simulink model "nmpc_sim_ee"  (R2022a)
settings: Solver=ode45  StartTime=0.0  StopTime=7  FixedStep=0.1  RelTol=1e-3
values from neighbouring files (symbols this model uses):
  N = n + 6    [ctrl_comp.m]    (also in nmpc_ee_2DoF.m; nmpc_ee_6DoF.m; nmpc_ee_subtest.m; nmpc_joint.m)
  ref = struct()    [nmpc_ee_2DoF.m]    (also in nmpc_ee_6DoF.m; nmpc_ee_subtest.m)
  Tp = 5    [nmpc_ee_2DoF.m]    (also in nmpc_ee_6DoF.m; nmpc_ee_subtest.m; nmpc_joint.m = 10)
  Ts = 0.1    [nmpc_ee_2DoF.m]    (also in nmpc_ee_6DoF.m; nmpc_ee_subtest.m = 0.5; nmpc_joint.m = 0.2)
  xee0 = [xee0; zeros(3, 1)]    [nmpc_ee_2DoF.m]    (also in nmpc_ee_6DoF.m = [xee0; psi_ee]; nmpc_ee_subtest.m = xee_start)
libraries: mpclib x1
settings Model: Creator=charl  LastModifiedBy=charl

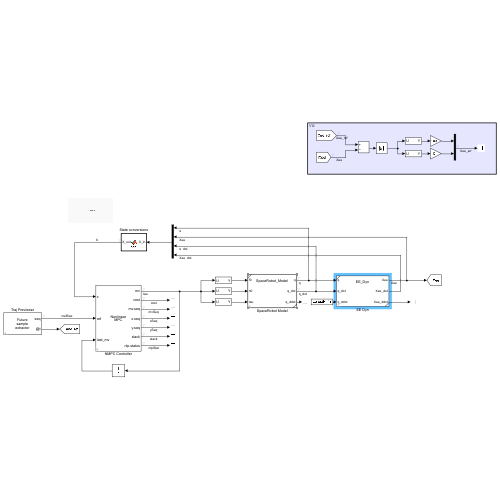
[thumbnail: Simulink's stored preview of the top-level diagram]
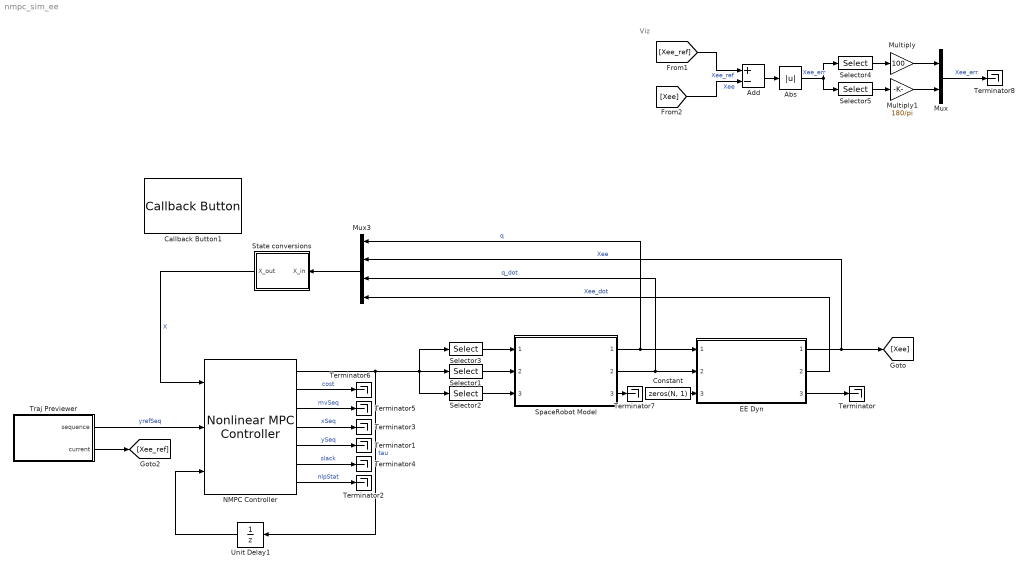
== system nmpc_sim_ee ==
  note: Viz
  Abs : Abs  SaturateOnIntegerOverflow=off
  Add : Sum  Inputs=+-
  Callback Button1 : CallbackButton  ButtonText=Animate results
      settings: ClickFcn=|
      | close all
      | try
      |     sr.animate(out.q, 'fps', 17, 'rate', 1);
      | catch
      |     close all
      | end
  Constant : Constant  Value=zeros(N, 1)
  EE Dyn : Subsystem  ReferencedSubsystem=EE_Dyn  spaceRobot=sr  Xee0=xee0.'
  Multiply : Gain  Gain=100
  Multiply1 : Gain  Gain=180/pi
  Mux : Mux  Inputs=2
  Mux3 : Mux
  NMPC Controller : mpclib/Nonlinear MPC Controller  SCDEnableBlockLinearizationSpecification=on  nlmpcobj=nlmpc_ee  UseObjectTs=on  TsControl=Ts  UseMEX=off  mexname=nlmpc_ee_SR6_mex  md_enabled=off  mvtarget_enabled=off  param_enabled=off  cost_enabled=on  mvseq_enabled=on  stateseq_enabled=on  ovseq_enabled=on  slack_enabled=on  status_enabled=on  ov_min=off  ov_max=off  mv_min=off  mv_max=off  mvrate_min=off  mvrate_max=off  state_min=off  state_max=off  ov_weight=off  mv_weight=off  mvrate_weight=off  ecr_weight=off  nlp_initialize=off
  Selector1 : Selector  IndexOptions=Index vector (dialog)  Indices=[4:6]  OutputSizes=1
  Selector2 : Selector  IndexOptions=Index vector (dialog)  Indices=[7:N]  OutputSizes=1
  Selector3 : Selector  IndexOptions=Index vector (dialog)  Indices=[1:3]  OutputSizes=1
  Selector4 : Selector  IndexOptions=Index vector (dialog)  Indices=[1:3]  OutputSizes=1
  Selector5 : Selector  IndexOptions=Index vector (dialog)  Indices=[4:6]  OutputSizes=1
  SpaceRobot Model : Subsystem  ReferencedSubsystem=SpaceRobot_Model  spaceRobot=sr  jointCstr=off  q_0=q0  q_dot_0=q_dot_0
  State conversions : MATLAB Function  TreatAsAtomicUnit=on
  Terminator{,1..8} (9 alike) : Terminator
  Traj Previewer : Subsystem  mask{signal=ref, ts=Ts, steps=Tp}
      mask prompts: signal "Signal name"; ts "Sampling time"; steps "Number of previewing steps"
      mask init:
      | ts = evalin('base',get_param(gcbh,'ts'));
      | signal = evalin('base',get_param(gcbh,'signal'));
      | steps = evalin('base',get_param(gcbh,'steps'));
      | data = mpc_previewer_maskinit(signal,ts);
      mask Display:
      | fprintf('Future\nsample\nextractor');
      | port_label('output', 1, 'seq')
      | port_label('output', 2, '@t')
  Unit Delay1 : UnitDelay  SampleTime=-1  HasFrameUpgradeWarning=on
  wires:
  NMPC Controller/1 -> Unit Delay1/1, Selector2/1, Selector1/1, Selector3/1  "tau"
  Selector2/1 -> SpaceRobot Model/3
  Selector1/1 -> SpaceRobot Model/2
  Selector3/1 -> SpaceRobot Model/1
  Unit Delay1/1 -> NMPC Controller/3
  Traj Previewer/1(sequence) -> NMPC Controller/2  "yrefSeq"
  SpaceRobot Model/2 -> Mux3/3, EE Dyn/2  "q_dot"
  SpaceRobot Model/1 -> EE Dyn/1, Mux3/1  "q"
  [Xee_ref] -> Add/1  "Xee_ref"
  [Xee] -> Add/2  "Xee"
  State conversions/1(X_out) -> NMPC Controller/1  "X"
  EE Dyn/1 -> Mux3/2, [Xee]  "Xee"
  EE Dyn/2 -> Mux3/4  "Xee_dot"
  NMPC Controller/4 -> Terminator3/1  "xSeq"
  NMPC Controller/5 -> Terminator1/1  "ySeq"
  NMPC Controller/7 -> Terminator2/1  "nlpStat"
  Traj Previewer/2(current) -> [Xee_ref]
  NMPC Controller/6 -> Terminator4/1  "slack"
  NMPC Controller/2 -> Terminator6/1  "cost"
  NMPC Controller/3 -> Terminator5/1  "mvSeq"
  SpaceRobot Model/3 -> Terminator7/1
  EE Dyn/3 -> Terminator/1
  Constant/1 -> EE Dyn/3
  Add/1 -> Abs/1
  Mux/1 -> Terminator8/1  "Xee_err"
  Mux3/1 -> State conversions/1(X_in)
  Abs/1 -> Selector4/1, Selector5/1  "Xee_err"
  Selector4/1 -> Multiply/1
  Selector5/1 -> Multiply1/1
  Multiply/1 -> Mux/1
  Multiply1/1 -> Mux/2

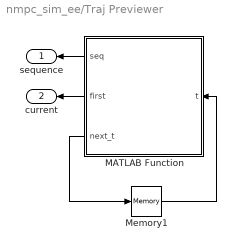
== system nmpc_sim_ee/Traj Previewer ==
  MATLAB Function : MATLAB Function  TreatAsAtomicUnit=on
  Memory1 : Memory  InheritSampleTime=on  LinearizeAsDelay=on
  sequence : Outport
  current : Outport  Port=2
  wires:
  MATLAB Function/1(seq) -> sequence/1
  MATLAB Function/2(first) -> current/1
  Memory1/1 -> MATLAB Function/1(t)
  MATLAB Function/3(next_t) -> Memory1/1

== matlab function nmpc_sim_ee/State conversions ==
  data: X_in input; X_out output; N parameter
function X_out = fcn(X_in, N)
% To converts q to x
% Input
%   X = [qb; qm; Xee; qb_dot; qm_dot; Xee_dot]
%       qb = [rx; ry; rx; psi_x; psi_y; psi_z] : Base coords
%       qm: Manip. coords
%       Xee = [rx_ee; ry_ee; rz_ee; psi_x_ee; psi_y_ee; psi_z_ee] : End-effector coords
%
%       qb_dot = [vx; vy; vz; wx; wy; wz]: Base velocities
%       qm_dot: Manip. joint rates
%       Xee_dot = [vx_ee; vy_ee; vz_ee; wx_ee; wy_ee; wz_ee]: End-effector velocities
%
% Output
%   X_out = [qb; qm; Xee; xb_dot; qm_dot; xee_dot]

q = X_in(1:N);
q_ee = X_in(N+1:N+6);

q_dot = X_in(N+7:2*N+6);
q_ee_dot = X_in(end-5:end);

X_out = X_in;

X_out(N+10:N+12) = omega2euler(q(4:6), q_dot(4:6)); % psi_b_dot = R_psi^-1*w_b

% X_out(end-2:end) = omega2euler(q_ee(4:6), q_ee_dot(4:6)); % psi_ee_dot = R_psi^-1*w_ee

== matlab function nmpc_sim_ee/Traj Previewer/MATLAB Function ==
  settings: updateMethod=DISCRETE  sampleTime=ts
  data: data parameter; seq output; steps parameter; t input; first output; next_t output
function [seq,first,next_t] = fcn(data,steps,t)
%#codegen
[seq,first,next_t] = mpcblock_preview('ref',data,steps,t);
